simulink model "tremolo2"  (R2025b)
settings: Solver=FixedStepDiscrete  StartTime=0.0  StopTime=inf  FixedStep=128/48000  RelTol=1e-3
model workspace (MATLAB code in the model file):
  | Gain_rt = Simulink.Parameter(1.0);
  | Bypass_rt = Simulink.Parameter(false);
settings Model: Creator=linogarciamorales  LastModifiedBy=linogarciamorales
settings OptimizationCC: EnhancedBackFolding=on  PassReuseOutputArgsAs=Individual arguments  ZeroExternalMemoryAtStartup=off  ZeroInternalMemoryAtStartup=off  OptimizeBlockOrder=speed  DifferentSizesBufferReuse=on  OptimizationCustomize=off  EfficientTunableParamExpr=on
settings DebuggingCC: ParameterTunabilityLossMsg=error
settings SFSimCC: MATLABDynamicMemAlloc=off
settings RTWCC: SystemTargetFile=ert.tlc  GenCodeOnly=on  TemplateMakefile=ert_default_tmf  Description=Embedded Coder
settings CodeAppCC: ForceParamTrailComments=on  IgnoreCustomStorageClasses=off  OperatorAnnotations=on  SimulinkDataObjDesc=on  SFDataObjDesc=on  InsertBlockDesc=on
settings ERTTargetCC: InlinedParameterPlacement=Hierarchical  ERTCustomFileTemplate=example_file_process.tlc  TargetLangStandard=C99 (ISO)  GenerateSampleERTMain=on  SupportNonInlinedSFcns=on

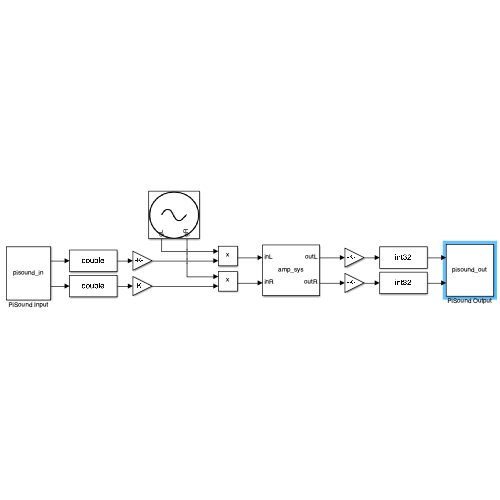
[thumbnail: Simulink's stored preview of the top-level diagram]
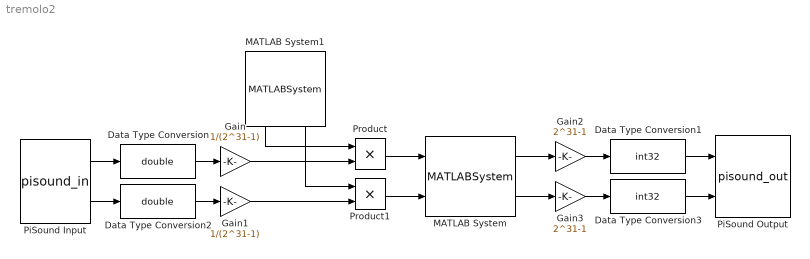
== system tremolo2 ==
  Data Type Conversion : DataTypeConversion  OutDataTypeStr=double  SaturateOnIntegerOverflow=off  RndMeth=Floor
  Data Type Conversion1 : DataTypeConversion  OutDataTypeStr=int32  SaturateOnIntegerOverflow=off  RndMeth=Floor
  Data Type Conversion2 : DataTypeConversion  OutDataTypeStr=double  SaturateOnIntegerOverflow=off  RndMeth=Floor
  Data Type Conversion3 : DataTypeConversion  OutDataTypeStr=int32  SaturateOnIntegerOverflow=off  RndMeth=Floor
  Gain : Gain  Gain=1/(2^31-1)
  Gain1 : Gain  Gain=1/(2^31-1)
  Gain2 : Gain  Gain=2^31-1
  Gain3 : Gain  Gain=2^31-1
  MATLAB System : MATLABSystem  System=amp_sys  Fs=48000  Gain=Gain_rt  Bypass=Bypass_rt  SimulateUsing=Code generation
      mask Type: amp_sys
  MATLAB System1 : MATLABSystem  System=lfo_sys  N=128  Fs=48000  Rate=5  Depth=0.8  StereoPhase=0  WaveSel=uint8( 1 )  SimulateUsing=Code generation
      mask Type: lfo_sys
  PiSound Input : S-Function  FunctionName=pisound_in  Parameters=48000, 128, 0  SFunctionDeploymentMode=off  EnableBusSupport=off
  PiSound Output : S-Function  FunctionName=pisound_out  Parameters=48000, 128, 0  SFunctionDeploymentMode=off  EnableBusSupport=off
  Product : Product  OutDataTypeStr=double
  Product1 : Product  OutDataTypeStr=double
  wires:
  PiSound Input/1 -> Data Type Conversion/1
  Data Type Conversion1/1 -> PiSound Output/1
  Data Type Conversion3/1 -> PiSound Output/2
  Gain2/1 -> Data Type Conversion1/1
  Gain3/1 -> Data Type Conversion3/1
  Data Type Conversion/1 -> Gain/1
  Data Type Conversion2/1 -> Gain1/1
  MATLAB System/1 -> Gain2/1
  MATLAB System/2 -> Gain3/1
  Gain/1 -> Product/2
  MATLAB System1/1 -> Product/1
  Product/1 -> MATLAB System/1
  MATLAB System1/2 -> Product1/1
  Gain1/1 -> Product1/2
  Product1/1 -> MATLAB System/2
  PiSound Input/2 -> Data Type Conversion2/1
